simulink model "threephase SAPF"  (R2024a)
settings: Solver=VariableStepAuto  StartTime=0  StopTime=1  MaxStep=1e-5  RelTol=1e-3
libraries: spsDiodeLib x6, spsIGBTDiodeLib x6, spsSeriesRLCBranchLib x3, spsThreePhaseSeriesRLCBranchLib x3, spsThreePhaseVIMeasurementLib x3, spsGroundLib x2, spsThreePhaseSourceLib x1, spsThreePhaseBreakerLib x1, spsVoltageMeasurementLib x1, sps_lib x1
settings Model: NumberOfSteps=5  PacingRate=0.710000  Creator=Zain  LastModifiedBy=Zain
settings SolverCC: ZeroCrossAlgorithm=Adaptive
settings DebuggingCC: MaskedZcDiagnostic=none

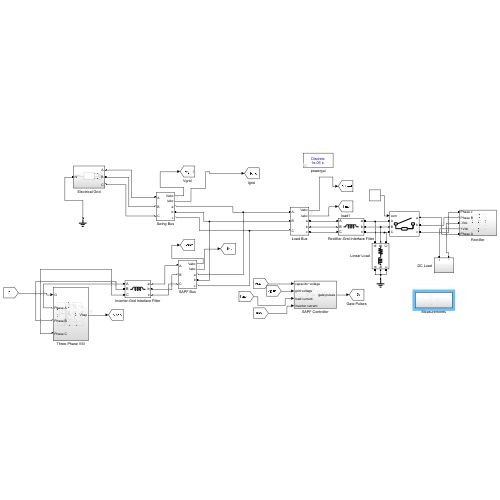
[thumbnail: Simulink's stored preview of the top-level diagram]
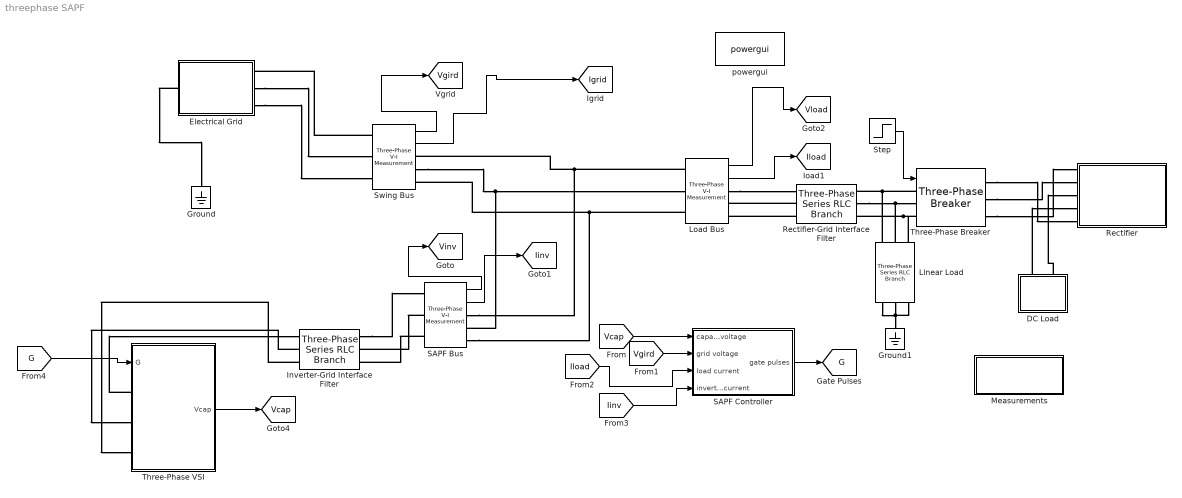
== system threephase SAPF ==
  DC Load : Subsystem
  Electrical Grid : Subsystem
  Ground : spsGroundLib/Ground  LConnTagsString=a
  Ground1 : spsGroundLib/Ground  LConnTagsString=a
  Inverter-Grid Interface Filter : spsThreePhaseSeriesRLCBranchLib/Three-Phase Series RLC Branch  LConnTagsString=A|B|C  RConnTagsString=A|B|C  BranchType=L  Resistance=1  Inductance=1e-3  Capacitance=1e-6  Measurements=None
  Linear Load : spsThreePhaseSeriesRLCBranchLib/Three-Phase Series RLC Branch  LConnTagsString=A|B|C  RConnTagsString=A|B|C  BranchType=RL  Resistance=10  Inductance=1e-3  Capacitance=1e-6  Measurements=None
  Load Bus : spsThreePhaseVIMeasurementLib/Three-Phase V-I Measurement  VoltageMeasurement=phase-to-ground  SetLabelV=off  LabelV=Vabc  Vpu=off  VpuLL=off  CurrentMeasurement=yes  SetLabelI=off  LabelI=Iabc  Ipu=off  Pbase=100e6  Vbase=500e3  OutputType=Complex  PhasorSimulation=off  PSBequivalent=0
  Measurements : Subsystem
  Rectifier : Subsystem
  Rectifier-Grid Interface Filter : spsThreePhaseSeriesRLCBranchLib/Three-Phase Series RLC Branch  LConnTagsString=A|B|C  RConnTagsString=A|B|C  BranchType=L  Resistance=0.25e-3  Inductance=1e-3  Capacitance=1e-6  Measurements=None
  SAPF Bus : spsThreePhaseVIMeasurementLib/Three-Phase V-I Measurement  VoltageMeasurement=phase-to-ground  SetLabelV=off  LabelV=Vabc  Vpu=off  VpuLL=off  CurrentMeasurement=yes  SetLabelI=off  LabelI=Iabc  Ipu=off  Pbase=100e6  Vbase=500e3  OutputType=Complex  PhasorSimulation=off  PSBequivalent=0
  SAPF Controller : Subsystem
  Step : Step  Time=0.5  SampleTime=0
  Swing Bus : spsThreePhaseVIMeasurementLib/Three-Phase V-I Measurement  VoltageMeasurement=phase-to-ground  SetLabelV=off  LabelV=Vabc  Vpu=off  VpuLL=off  CurrentMeasurement=yes  SetLabelI=off  LabelI=Iabc  Ipu=off  Pbase=100e6  Vbase=500e3  OutputType=Complex  PhasorSimulation=off  PSBequivalent=0
  Three-Phase Breaker : spsThreePhaseBreakerLib/Three-Phase Breaker  InitialState=open  SwitchA=on  SwitchB=on  SwitchC=on  SwitchTimes="[1/60  5/60]"  External=on  BreakerResistance=0.01  SnubberResistance=1e6  SnubberCapacitance=inf  Measurements=None
  Three-Phase VSI : Subsystem
  powergui : sps_lib/powergui  Priority=1  SimulationMode=Discrete  SampleTime=1e-5  frequency=60  Iterations=50  frequencyindice=50  Pbase=100e6  ErrMax=1e-4  UnitsV=kV  UnitsW=MW  buscounter=0  FunctionMessages=off  echomessages=off  EnableUseOfTLC=off  CurrentSourceSwitches=off  DisableSnubberDevices=off  DisableRonSwitches=off  DisableVfSwitches=off  DisplayEquations=off  AutomaticDiscreteSolvers=off  SolverType=Tustin/Backward Euler (TBE)  Interpol=off  ExternalGateDelay=off  methode=off  Ts=100  x0status=blocks  SPID=on  SwTol=0  HookPort=off  NonlinearTolerance=1e-4  nMaxIteration=100  ContinueOnMaxIteration=off  RestoreLinks=warning  ResistiveCurrentMeasurement=off  Frange=[0:2:500]  Ylog=off  Xlog=on  ShowGrid=off  save=off  variable=ZData  structure=0  ZoomFFT=off  StartTime=0.0  cycles=1  DisplayStyle=1  fundamental=60  FreqAxis=off  MaxFrequency=1000  frequencyindicesteady=1  RmsSteady=1  display=off
  tag scope: G=global, Igrid=global, Iinv=global, Iload=global, Vcap=global, Vgird=global, Vinv=global, Vload=global
  wires:
  Swing Bus/2 -> [Igrid]
  Swing Bus/1 -> [Vgird]
  SAPF Bus/1 -> [Vinv]
  SAPF Bus/2 -> [Iinv]
  Load Bus/1 -> [Vload]
  Load Bus/2 -> [Iload]
  Step/1 -> Three-Phase Breaker/1
  Three-Phase VSI/1(Vcap) -> [Vcap]
  SAPF Controller/1(gate pulses) -> [G]
  [G] -> Three-Phase VSI/1(G)
  [Vcap] -> SAPF Controller/1(capacitor voltage)
  [Vgird] -> SAPF Controller/2(grid voltage)
  [Iload] -> SAPF Controller/3(load current)
  [Iinv] -> SAPF Controller/4(inverter current)
  connections:
  Electrical Grid/LConn1 -- Ground/LConn1
  Swing Bus/LConn1 -- Electrical Grid/RConn1
  Electrical Grid/RConn2 -- Swing Bus/LConn2
  Electrical Grid/RConn3 -- Swing Bus/LConn3
  Load Bus/RConn1 -- Rectifier-Grid Interface Filter/LConn1
  Rectifier-Grid Interface Filter/LConn2 -- Load Bus/RConn2
  Rectifier-Grid Interface Filter/LConn3 -- Load Bus/RConn3
  Three-Phase Breaker/LConn1 -- Linear Load/LConn1 -- Rectifier-Grid Interface Filter/RConn1
  Rectifier-Grid Interface Filter/RConn2 -- Linear Load/LConn2 -- Three-Phase Breaker/LConn2
  Three-Phase Breaker/LConn3 -- Linear Load/LConn3 -- Rectifier-Grid Interface Filter/RConn3
  Linear Load/RConn1 -- Linear Load/RConn3 -- Ground1/LConn1 -- Linear Load/RConn2
  Three-Phase VSI/LConn1 -- Inverter-Grid Interface Filter/LConn1
  Inverter-Grid Interface Filter/LConn2 -- Three-Phase VSI/LConn2
  Inverter-Grid Interface Filter/LConn3 -- Three-Phase VSI/LConn3
  DC Load/LConn2 -- Rectifier/LConn3
  DC Load/LConn1 -- Rectifier/LConn4
  Three-Phase Breaker/RConn1 -- Rectifier/LConn5
  Three-Phase Breaker/RConn2 -- Rectifier/LConn2
  Three-Phase Breaker/RConn3 -- Rectifier/LConn1
  Load Bus/LConn1 -- SAPF Bus/RConn1 -- Swing Bus/RConn1
  Swing Bus/RConn2 -- SAPF Bus/RConn2 -- Load Bus/LConn2
  Load Bus/LConn3 -- SAPF Bus/RConn3 -- Swing Bus/RConn3
  Inverter-Grid Interface Filter/RConn1 -- SAPF Bus/LConn1
  SAPF Bus/LConn2 -- Inverter-Grid Interface Filter/RConn2
  SAPF Bus/LConn3 -- Inverter-Grid Interface Filter/RConn3

== system threephase SAPF/DC Load ==
  Series RLC Branch : spsSeriesRLCBranchLib/Series RLC Branch  LConnTagsString=__new0  RConnTagsString=__new0  BranchType=R  Resistance=6.5  Inductance=1e-3  SetiL0=off  InitialCurrent=0  Capacitance=1e-6  Setx0=off  InitialVoltage=0  Measurements=None
  Series RLC Branch1 : spsSeriesRLCBranchLib/Series RLC Branch  LConnTagsString=__new0  RConnTagsString=__new0  BranchType=L  Resistance=1  Inductance=20e-3  SetiL0=off  InitialCurrent=0  Capacitance=1e-6  Setx0=off  InitialVoltage=0  Measurements=None
  + : PMIOPort  Side=Left
  - : PMIOPort  Port=2  Side=Left
  connections:
  Series RLC Branch/LConn1 -- Series RLC Branch1/RConn1
  -/RConn1 -- Series RLC Branch/RConn1
  +/RConn1 -- Series RLC Branch1/LConn1

== system threephase SAPF/Electrical Grid ==
  Three-Phase Source : spsThreePhaseSourceLib/Three-Phase Source  InternalConnection=Yn  VoltagePhases=off  Voltage=220*sqrt(3)  PhaseAngle=0  Voltage_phases=[25e3 25e3 25e3]/sqrt(3)  PhaseAngles_phases=[0 -120 +120]  Frequency=50  NonIdealSource=on  SpecifyImpedance=on  Resistance=0.8929  Inductance=16.58e-3  ShortCircuitLevel=100e6  BaseVoltage=25e3  XRratio=7  BusType=swing  Pref=10e3  Qref=0  Prefabc=[10e3, 10e3, 10e3]  Qrefabc=[0, 0, 0]  Qmin=-inf  Qmax=inf
  A : PMIOPort  Side=Right
  B : PMIOPort  Port=2  Side=Right
  C : PMIOPort  Port=3  Side=Right
  N : PMIOPort  Port=4  Side=Left
  connections:
  Three-Phase Source/LConn1 -- N/RConn1
  Three-Phase Source/RConn3 -- C/RConn1
  Three-Phase Source/RConn2 -- B/RConn1
  Three-Phase Source/RConn1 -- A/RConn1

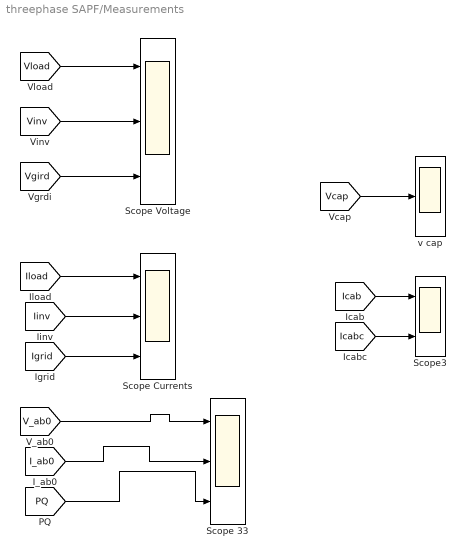
== system threephase SAPF/Measurements ==
  Scope 33 : Scope  NumInputPorts=3
  Scope Currents : Scope  NumInputPorts=3
  Scope Voltage : Scope  NumInputPorts=3
  Scope3 : Scope  NumInputPorts=2
  v cap : Scope
  wires:
  [Vload] -> Scope Voltage/1
  [Vinv] -> Scope Voltage/2
  [Vgird] -> Scope Voltage/3
  [Iload] -> Scope Currents/1
  [Iinv] -> Scope Currents/2
  [PQ] -> Scope 33/3
  [I_ab0] -> Scope 33/2
  [V_ab0] -> Scope 33/1
  [Vcap] -> v cap/1
  [Icab] -> Scope3/1
  [Icabc] -> Scope3/2
  [Igrid] -> Scope Currents/3

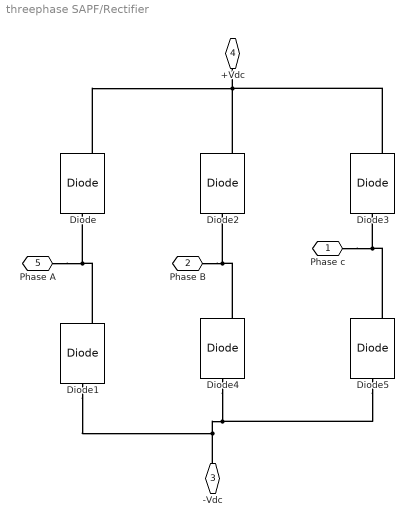
== system threephase SAPF/Rectifier ==
  Diode{,1..5} (6 alike) : spsDiodeLib/Diode  Ron=0.001  Lon=0  Vf=0.8  IC=0  UseSnubber=0  Rs=1e4  Cs=0.1e-6  Measurements=on
  Phase c : PMIOPort  Side=Left
  Phase B : PMIOPort  Port=2  Side=Left
  -Vdc : PMIOPort  Port=3  Side=Left
  +Vdc : PMIOPort  Port=4  Side=Left
  Phase A : PMIOPort  Port=5  Side=Left
  connections:
  Diode3/RConn1 -- Diode/RConn1 -- +Vdc/RConn1 -- Diode2/RConn1
  Phase B/RConn1 -- Diode4/RConn1 -- Diode2/LConn1
  Phase c/RConn1 -- Diode5/RConn1 -- Diode3/LConn1
  Phase A/RConn1 -- Diode1/RConn1 -- Diode/LConn1
  -Vdc/RConn1 -- Diode1/LConn1 -- Diode4/LConn1 -- Diode5/LConn1

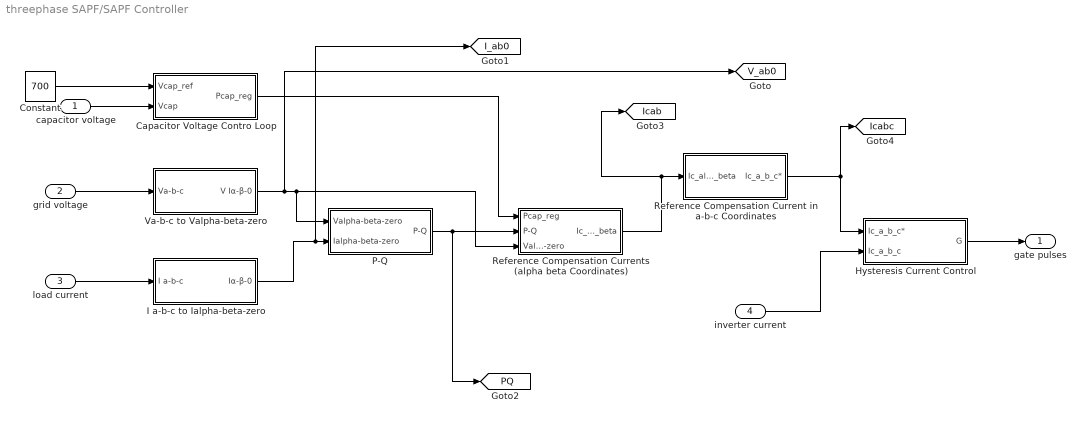
== system threephase SAPF/SAPF Controller ==
  capacitor voltage : Inport
  grid voltage : Inport  Port=2
  load current : Inport  Port=3
  inverter current : Inport  Port=4
  Capacitor Voltage Contro Loop : Subsystem
  Constant : Constant  Value=700
  Hysteresis Current Control : Subsystem
  I a-b-c to Ialpha-beta-zero : Subsystem
  P-Q : Subsystem
  Reference Compensation Current in a-b-c Coordinates : Subsystem
  Reference Compensation Currents (alpha beta Coordinates) : Subsystem
  Va-b-c to Valpha-beta-zero : Subsystem
  gate pulses : Outport
  tag scope: I_ab0=global, Icab=global, Icabc=global, PQ=global, V_ab0=global
  wires:
  grid voltage/1 -> Va-b-c to Valpha-beta-zero/1(Va-b-c)
  load current/1 -> I a-b-c to Ialpha-beta-zero/1(I a-b-c)
  Constant/1 -> Capacitor Voltage Contro Loop/1(Vcap_ref)
  capacitor voltage/1 -> Capacitor Voltage Contro Loop/2(Vcap)
  I a-b-c to Ialpha-beta-zero/1(Iα-β-0) -> [I_ab0], P-Q/2(Ialpha-beta-zero)
  Va-b-c to Valpha-beta-zero/1(V Iα-β-0) -> [V_ab0], Reference Compensation Currents (alpha beta Coordinates)/3(Valpha-beta-zero), P-Q/1(Valpha-beta-zero)
  P-Q/1(P-Q) -> Reference Compensation Currents (alpha beta Coordinates)/2(P-Q), [PQ]
  Capacitor Voltage Contro Loop/1(Pcap_reg) -> Reference Compensation Currents (alpha beta Coordinates)/1(Pcap_reg)
  Reference Compensation Currents (alpha beta Coordinates)/1("Ic_alpha_beta ") -> [Icab], Reference Compensation Current in a-b-c Coordinates/1(Ic_alpha_beta)
  Reference Compensation Current in a-b-c Coordinates/1(Ic_a_b_c*) -> [Icabc], Hysteresis Current Control/1(Ic_a_b_c*)
  inverter current/1 -> Hysteresis Current Control/2(Ic_a_b_c)
  Hysteresis Current Control/1(G) -> gate pulses/1

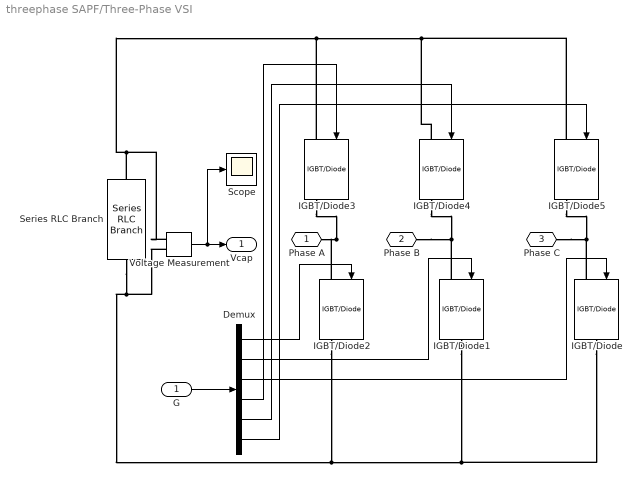
== system threephase SAPF/Three-Phase VSI ==
  G : Inport
  Demux : Demux  Outputs=6
  IGBT/Diode : spsIGBTDiodeLib/IGBT//Diode  Ron=1e-3  Rs=1e5  Cs=inf  Measurements=off
  IGBT/Diode1 : spsIGBTDiodeLib/IGBT//Diode  Ron=1e-3  Rs=1e5  Cs=inf  Measurements=off
  IGBT/Diode{2..5} (4 alike) : spsIGBTDiodeLib/IGBT//Diode  Ron=1e-3  Rs=1e5  Cs=inf  Measurements=on
  Scope : Scope
  Series RLC Branch : spsSeriesRLCBranchLib/Series RLC Branch  LConnTagsString=__new0  RConnTagsString=__new0  BranchType=C  Resistance=1  Inductance=1e-3  SetiL0=off  InitialCurrent=0  Capacitance=1e-3  Setx0=on  InitialVoltage=700  Measurements=Branch voltage
  Voltage Measurement : spsVoltageMeasurementLib/Voltage Measurement  PhasorSimulation=off  OutputType=Complex  PSBequivalent=0
  Phase A : PMIOPort  Side=Left
  Phase B : PMIOPort  Port=2  Side=Left
  Phase C : PMIOPort  Port=3  Side=Left
  Vcap : Outport
  wires:
  Voltage Measurement/1 -> Scope/1, Vcap/1
  G/1 -> Demux/1
  Demux/1 -> IGBT/Diode2/1
  Demux/2 -> IGBT/Diode1/1
  Demux/3 -> IGBT/Diode/1
  Demux/4 -> IGBT/Diode3/1
  Demux/5 -> IGBT/Diode4/1
  Demux/6 -> IGBT/Diode5/1
  connections:
  IGBT/Diode2/RConn1 -- Series RLC Branch/RConn1 -- Voltage Measurement/LConn2 -- IGBT/Diode1/RConn1 -- IGBT/Diode/RConn1
  Phase B/RConn1 -- IGBT/Diode4/RConn1 -- IGBT/Diode1/LConn1
  Phase C/RConn1 -- IGBT/Diode5/RConn1 -- IGBT/Diode/LConn1
  Phase A/RConn1 -- IGBT/Diode3/RConn1 -- IGBT/Diode2/LConn1
  Voltage Measurement/LConn1 -- IGBT/Diode3/LConn1 -- IGBT/Diode4/LConn1 -- IGBT/Diode5/LConn1 -- Series RLC Branch/LConn1

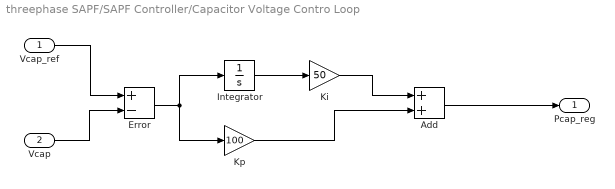
== system threephase SAPF/SAPF Controller/Capacitor Voltage Contro Loop ==
  Vcap_ref : Inport
  Vcap : Inport  Port=2
  Add : Sum
  Error : Sum  Inputs=+-
  Integrator : Integrator
  Ki : Gain  Gain=50
  Kp : Gain  Gain=100
  Pcap_reg : Outport
  wires:
  Vcap/1 -> Error/2
  Error/1 -> Integrator/1, Kp/1
  Kp/1 -> Add/2
  Integrator/1 -> Ki/1
  Ki/1 -> Add/1
  Add/1 -> Pcap_reg/1
  Vcap_ref/1 -> Error/1

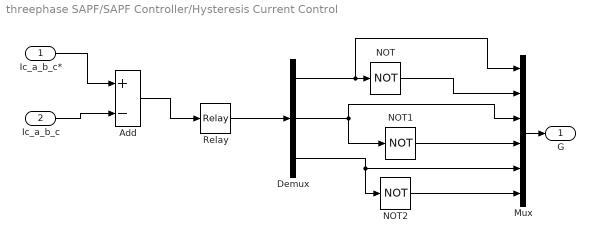
== system threephase SAPF/SAPF Controller/Hysteresis Current Control ==
  Ic_a_b_c* : Inport
  Ic_a_b_c : Inport  Port=2
  Add : Sum  Inputs=+-
  Demux : Demux  Outputs=3
  Mux : Mux  Inputs=6
  NOT : Logic  Operator=NOT  IconShape=distinctive  AllPortsSameDT=off  OutDataTypeStr=boolean
  NOT1 : Logic  Operator=NOT  IconShape=distinctive  AllPortsSameDT=off  OutDataTypeStr=boolean
  NOT2 : Logic  Operator=NOT  IconShape=distinctive  AllPortsSameDT=off  OutDataTypeStr=boolean
  Relay : Relay  OnSwitchValue=0.05  OffSwitchValue=-0.05  OutDataTypeStr=boolean  ZeroCross=off
  G : Outport
  wires:
  Ic_a_b_c*/1 -> Add/1
  Ic_a_b_c/1 -> Add/2
  Add/1 -> Relay/1
  Relay/1 -> Demux/1
  Demux/1 -> Mux/1, NOT/1
  Demux/2 -> NOT1/1, Mux/3
  Demux/3 -> NOT2/1, Mux/5
  NOT2/1 -> Mux/6
  NOT1/1 -> Mux/4
  NOT/1 -> Mux/2
  Mux/1 -> G/1

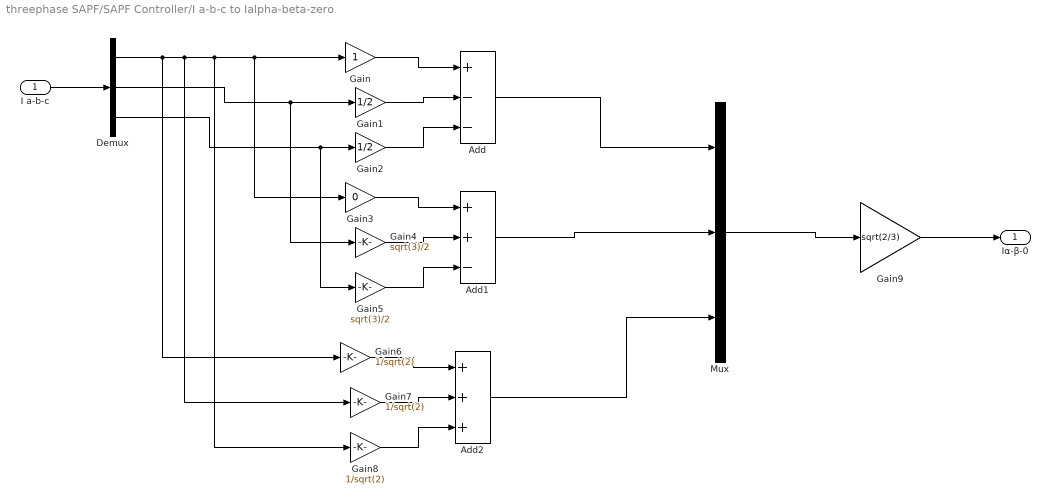
== system threephase SAPF/SAPF Controller/I a-b-c to Ialpha-beta-zero ==
  I a-b-c : Inport
  Add : Sum  Inputs=+--
  Add1 : Sum  Inputs=++-
  Add2 : Sum  Inputs=+++
  Demux : Demux  Outputs=3
  Gain : Gain
  Gain1 : Gain  Gain=1/2
  Gain2 : Gain  Gain=1/2
  Gain3 : Gain  Gain=0
  Gain4 : Gain  Gain=sqrt(3)/2
  Gain5 : Gain  Gain=sqrt(3)/2
  Gain6 : Gain  Gain=1/sqrt(2)
  Gain7 : Gain  Gain=1/sqrt(2)
  Gain8 : Gain  Gain=1/sqrt(2)
  Gain9 : Gain  Gain=sqrt(2/3)
  Mux : Mux  Inputs=3
  Iα-β-0 : Outport
  wires:
  I a-b-c/1 -> Demux/1
  Demux/1 -> Gain6/1, Gain7/1, Gain8/1, Gain3/1, Gain/1
  Demux/2 -> Gain1/1, Gain4/1
  Demux/3 -> Gain2/1, Gain5/1
  Gain/1 -> Add/1
  Gain1/1 -> Add/2
  Gain2/1 -> Add/3
  Gain4/1 -> Add1/2
  Gain3/1 -> Add1/1
  Gain5/1 -> Add1/3
  Gain7/1 -> Add2/2
  Gain6/1 -> Add2/1
  Gain8/1 -> Add2/3
  Add/1 -> Mux/1
  Add1/1 -> Mux/2
  Add2/1 -> Mux/3
  Mux/1 -> Gain9/1
  Gain9/1 -> Iα-β-0/1

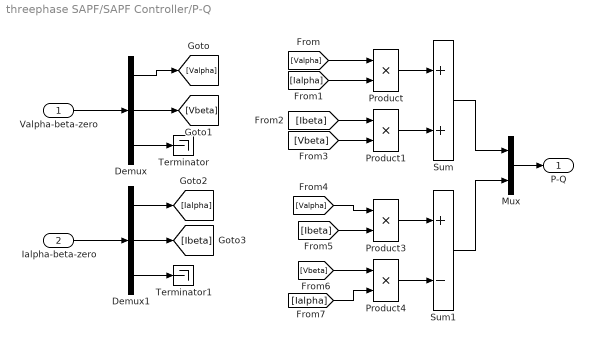
== system threephase SAPF/SAPF Controller/P-Q ==
  Valpha-beta-zero : Inport
  Ialpha-beta-zero : Inport  Port=2
  Demux : Demux  Outputs=3
  Demux1 : Demux  Outputs=3
  Mux : Mux  Inputs=2
  Product{,1,3..4} (4 alike) : Product
  Sum : Sum
  Sum1 : Sum  Inputs=+-
  Terminator : Terminator
  Terminator1 : Terminator
  P-Q : Outport
  wires:
  [Vbeta] -> Product4/1
  [Valpha] -> Product3/1
  Valpha-beta-zero/1 -> Demux/1
  [Vbeta] -> Product1/2
  Product3/1 -> Sum1/1
  Product4/1 -> Sum1/2
  Mux/1 -> P-Q/1
  [Ibeta] -> Product1/1
  Product1/1 -> Sum/2
  Demux/2 -> [Vbeta]
  Product/1 -> Sum/1
  [Ialpha] -> Product4/2
  Demux1/3 -> Terminator1/1
  Demux1/1 -> [Ialpha]
  [Ialpha] -> Product/2
  [Ibeta] -> Product3/2
  Demux/1 -> [Valpha]
  [Valpha] -> Product/1
  Demux1/2 -> [Ibeta]
  Demux/3 -> Terminator/1
  Ialpha-beta-zero/1 -> Demux1/1
  Sum/1 -> Mux/1
  Sum1/1 -> Mux/2

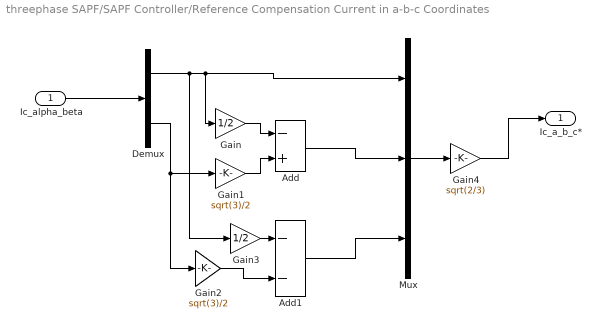
== system threephase SAPF/SAPF Controller/Reference Compensation Current in a-b-c Coordinates ==
  Ic_alpha_beta : Inport
  Add : Sum  Inputs=-+
  Add1 : Sum  Inputs=--
  Demux : Demux  Outputs=2
  Gain : Gain  Gain=1/2
  Gain1 : Gain  Gain=sqrt(3)/2
  Gain2 : Gain  Gain=sqrt(3)/2
  Gain3 : Gain  Gain=1/2
  Gain4 : Gain  Gain=sqrt(2/3)
  Mux : Mux  Inputs=3
  Ic_a_b_c* : Outport
  wires:
  Ic_alpha_beta/1 -> Demux/1
  Demux/1 -> Gain3/1, Gain/1, Mux/1
  Add1/1 -> Mux/3
  Add/1 -> Mux/2
  Gain/1 -> Add/1
  Gain1/1 -> Add/2
  Gain3/1 -> Add1/1
  Gain2/1 -> Add1/2
  Demux/2 -> Gain1/1, Gain2/1
  Mux/1 -> Gain4/1
  Gain4/1 -> Ic_a_b_c*/1

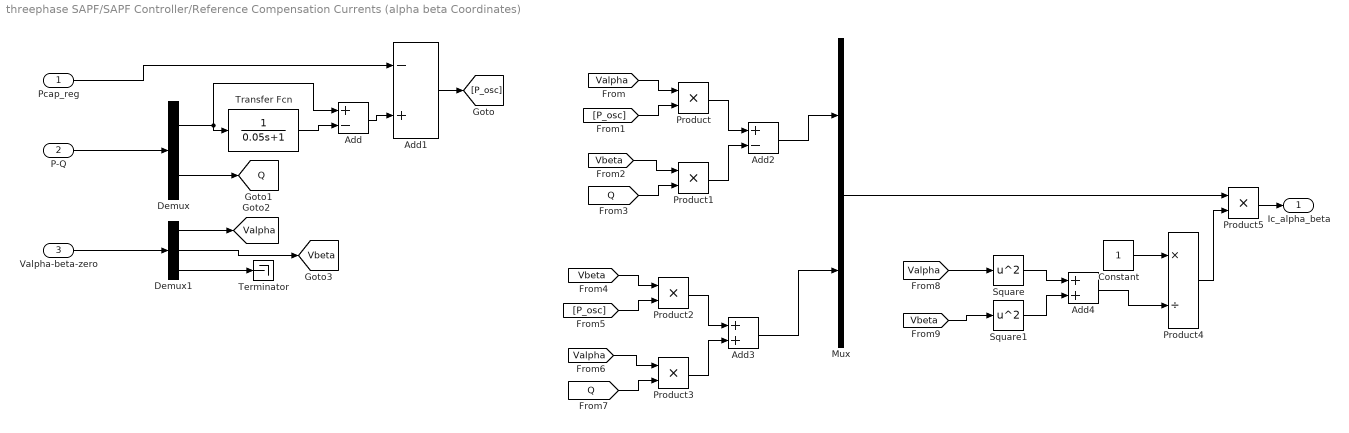
== system threephase SAPF/SAPF Controller/Reference Compensation Currents (alpha beta Coordinates) ==
  Pcap_reg : Inport
  P-Q : Inport  Port=2
  Valpha-beta-zero : Inport  Port=3
  Add : Sum  Inputs=+-
  Add1 : Sum  Inputs=-+
  Add2 : Sum  Inputs=+-
  Add3 : Sum
  Add4 : Sum
  Constant : Constant
  Demux : Demux  Outputs=2
  Demux1 : Demux  Outputs=3
  Mux : Mux  Inputs=2
  Product{,1..3,5} (5 alike) : Product
  Product4 : Product  Inputs=*/
  Square : Math  Operator=square
  Square1 : Math  Operator=square
  Terminator : Terminator
  Transfer Fcn : TransferFcn  Denominator=[0.05 1]
  "Ic_alpha_beta " : Outport
  tag scope: Q=global, Valpha=global, Vbeta=global
  wires:
  P-Q/1 -> Demux/1
  Valpha-beta-zero/1 -> Demux1/1
  Demux1/3 -> Terminator/1
  Demux/1 -> Add/1, Transfer Fcn/1
  Transfer Fcn/1 -> Add/2
  Pcap_reg/1 -> Add1/1
  Add/1 -> Add1/2
  Demux/2 -> [Q]
  Demux1/2 -> [Vbeta]
  Demux1/1 -> [Valpha]
  [Vbeta] -> Product1/1
  [Q] -> Product1/2
  [Valpha] -> Product/1
  [P_osc] -> Product/2
  Product/1 -> Add2/1
  Product1/1 -> Add2/2
  Add2/1 -> Mux/1
  [P_osc] -> Product2/2
  [Q] -> Product3/2
  Product3/1 -> Add3/2
  [Vbeta] -> Product2/1
  Product2/1 -> Add3/1
  [Valpha] -> Product3/1
  Add3/1 -> Mux/2
  [Valpha] -> Square/1
  [Vbeta] -> Square1/1
  Square1/1 -> Add4/2
  Square/1 -> Add4/1
  Add4/1 -> Product4/2
  Constant/1 -> Product4/1
  Mux/1 -> Product5/1
  Product4/1 -> Product5/2
  Product5/1 -> "Ic_alpha_beta "/1
  Add1/1 -> [P_osc]

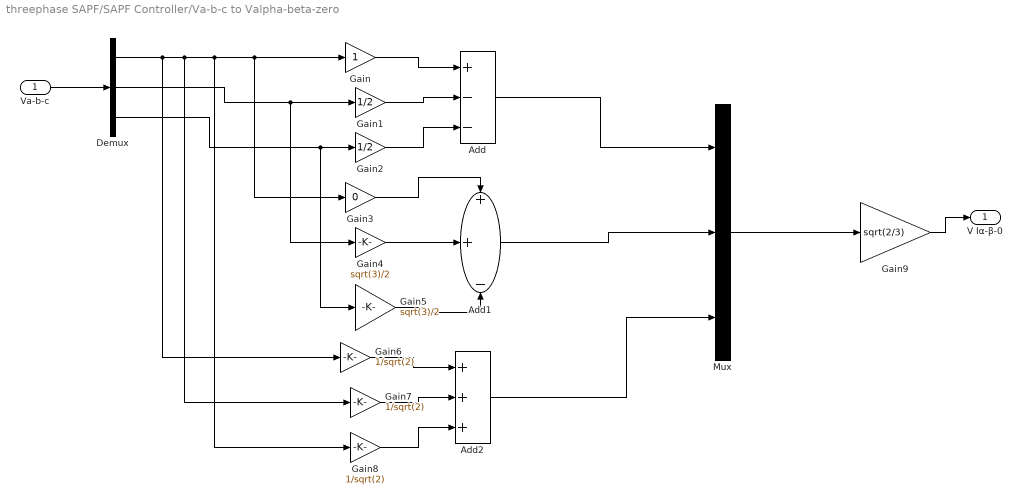
== system threephase SAPF/SAPF Controller/Va-b-c to Valpha-beta-zero ==
  Va-b-c : Inport
  Add : Sum  Inputs=+--
  Add1 : Sum  Inputs=++-
  Add2 : Sum  Inputs=+++
  Demux : Demux  Outputs=3
  Gain : Gain
  Gain1 : Gain  Gain=1/2
  Gain2 : Gain  Gain=1/2
  Gain3 : Gain  Gain=0
  Gain4 : Gain  Gain=sqrt(3)/2
  Gain5 : Gain  Gain=sqrt(3)/2
  Gain6 : Gain  Gain=1/sqrt(2)
  Gain7 : Gain  Gain=1/sqrt(2)
  Gain8 : Gain  Gain=1/sqrt(2)
  Gain9 : Gain  Gain=sqrt(2/3)
  Mux : Mux  Inputs=3
  V Iα-β-0 : Outport
  wires:
  Va-b-c/1 -> Demux/1
  Demux/1 -> Gain6/1, Gain7/1, Gain8/1, Gain3/1, Gain/1
  Demux/2 -> Gain1/1, Gain4/1
  Demux/3 -> Gain2/1, Gain5/1
  Gain/1 -> Add/1
  Gain1/1 -> Add/2
  Gain2/1 -> Add/3
  Gain4/1 -> Add1/2
  Gain3/1 -> Add1/1
  Gain5/1 -> Add1/3
  Gain7/1 -> Add2/2
  Gain6/1 -> Add2/1
  Gain8/1 -> Add2/3
  Add/1 -> Mux/1
  Add1/1 -> Mux/2
  Add2/1 -> Mux/3
  Mux/1 -> Gain9/1
  Gain9/1 -> V Iα-β-0/1
